simulink model "UGV"  (R2021b)
settings: Solver=VariableStepAuto  StartTime=0.0  StopTime=20  RelTol=1e-5
PreLoadFcn:
  | % initialize variables
  | initializeUnicycleModel;
undefined symbols (not defined in the file): ctrl, unicycle
settings Model: Creator=beniamino  LastModifiedBy=gioel
settings SolverCC: ZeroCrossAlgorithm=Adaptive
settings DataIOCC: InitialState=cartesianInitialStates  SaveFormat=Structure
settings DebuggingCC: IgnoredZcDiagnostic=none

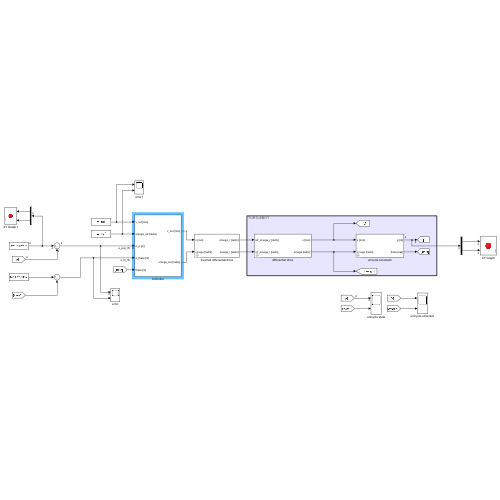
[thumbnail: Simulink's stored preview of the top-level diagram]
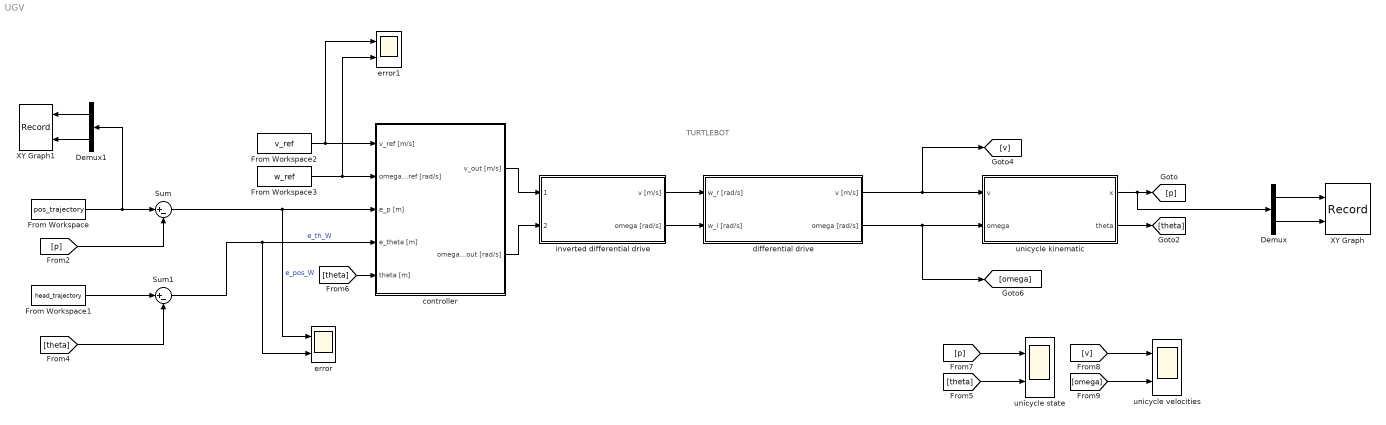
== system UGV ==
  note: TURTLEBOT
  Demux : Demux  Outputs=2
  Demux1 : Demux  Outputs=2
  From Workspace : FromWorkspace  VariableName=pos_trajectory
  From Workspace1 : FromWorkspace  VariableName=head_trajectory
  From Workspace2 : FromWorkspace  VariableName=v_ref
  From Workspace3 : FromWorkspace  VariableName=w_ref
  Sum : Sum  Inputs=|+-
  Sum1 : Sum  Inputs=|+-
  XY Graph : Record  FileSettingsInternal="{\"entries\":[{\"content\":{\"excelSettings\":{\"content\":{},\"type\":\"Streamout.ExcelSettings\"}},\"type\":\"Streamout.FileSettingStorage\",\"uuid\":\"13f76de6-499c-4140-b892-1cff53560195\"}],\"packageUris\":[\"http://schema.mathworks.com/mf0/streamout_blocks/R2020a\"],\"version\":\"1.0\"}"  Layout=[1 1]  SignalsInternal="{\"entries\":[{\"content\":{\"signals\":[{\"content\":{\"blockPath\":[\"UGV/XY Graph\"],\"channel\":[],\"dimensions\":[2],\"domain\":\"UGV/XY Graph\",\"hasChildren\":true,\"lineColor\":\"#77ac30\",\"plots\":[],\"port\":1,\"sid\":[\"\"],\"signalID\":231,\"signalName\":\"Mux\"},\"type\":\"RecordBlkView.Signal\",\"uuid\":\"fc620e12-1068-425f-97ba-d7612e3bfc5b\"},{\"content\":{\"blockPath\":[\"UGV/XY Graph\"],\"channel\":[1],\"dimensions\":[2],\"domain\":\"UGV/XY Graph\",\"lineColor\":\"#22b573\",\"parentID\":231,\"plots\":[],\"port\":1,\"sid\":[\"\"],\"signalID\":232,\"signalName\":\"Mux\"},\"type\":\"RecordBlkView.Signal\",\"uuid\":\"68e69acf-f8ce-4302-af24-f78098d05fbc\"},{\"content\":{\"blockPath\":[\"UGV/XY Graph\"],\"channel\":[],\"dimensions\":[2],\"domain\":\"UGV/XY Graph\",\"hasChildren\":true,\"lineColor\":\"#a2142f\",\"plots\":[],\"port\":2,\"sid\":[\"\"],\"signalID\":236,\"signalName\":\"Mux1\"},\"type\":\"RecordBlkView.Signal\",\"uuid\":\"04ece26b-ae12-44e9-b04e-33a75d772337\"},{\"content\":{\"blockPath\":[\"UGV/XY Graph\"],\"channel\":[1],\"dimensions\":[2],\"domain\":\"UGV/XY Graph\",\"lineColor\":\"#d95319\",\"parentID\":236,\"plots\":[],\"port\":2,\"sid\":[\"\"],\"signalID\":237,\"signalName\":\"Mux1\"},\"type\":\"RecordBlkView.Signal\",\"uuid\":\"c9d8e2c4-8b9b-40cc-9608-f78b40cf16be\"},{\"content\":{\"blockPath\":[\"UGV/XY Graph\"],\"channel\":[2],\"dimensions\":[2],\"domain\":\"UGV/XY Graph\",\"lineColor\":\"#edb120\",\"parentID\":231,\"plots\":[],\"port\":1,\"sid\":[\"\"],\"signalID\":240,\"signalName\":\"Mux\"},\"type\":\"RecordBlkView.Signal\",\"uuid\":\"41f5023c-efaf-446b-89f3-def201b5f8a6\"},{\"content\":{\"blockPath\":[\"UGV/XY Graph\"],\"channel\":[2],\"dimensions\":[2],\"domain\":\"UGV/XY Graph\",\"lineColor\":\"#7e2f8e\",\"parentID\":236,\"plots\":[],\"port\":2,\"sid\":[\"\"],\"signalID\":241,\"signalName\":\"Mux1\"},\"type\":\"RecordBlkView.Signal\",\"uuid\":\"77807980-b3eb-4829-a033-1b0bab4bfe93\"}]},\"type\":\"RecordBlkView.InputSignals\",\"uuid\":\"96da7dc8-515b-4996-b558-6921bb10ee03\"}],\"packageUris\":[\"http://schema.mathworks.com/mf0/streamout_blocks/R2020a\"],\"version\":\"1.0\"}"  VisualizationBindings="{\"xyplotplugin\":{\"info\":[{\"series\":[],\"subplotID\":1}]}}"  CompatibilityTag=XY
  XY Graph1 : Record  FileSettingsInternal="{\"entries\":[{\"content\":{\"excelSettings\":{\"content\":{},\"type\":\"Streamout.ExcelSettings\"}},\"type\":\"Streamout.FileSettingStorage\",\"uuid\":\"96a30333-0ed4-4420-9fea-70885ab511f6\"}],\"packageUris\":[\"http://schema.mathworks.com/mf0/streamout_blocks/R2020a\"],\"version\":\"1.0\"}"  Layout=[1 1]  SignalsInternal="{\"entries\":[{\"content\":{\"signals\":[]},\"type\":\"RecordBlkView.InputSignals\",\"uuid\":\"79161730-7756-4a65-8139-4cac527f2b4f\"}],\"packageUris\":[\"http://schema.mathworks.com/mf0/streamout_blocks/R2020a\"],\"version\":\"1.0\"}"  VisualizationBindings="{\"xyplotplugin\":{\"info\":[{\"series\":[{\"bindingParametersList\":[{\"parameter\":\"X-Axis\",\"signalID\":181,\"signalName\":\"Demux1:1\"},{\"parameter\":\"Y-Axis\",\"signalID\":185,\"signalName\":\"Demux1:2\"}],\"seriesID\":31783}],\"subplotID\":1}]}}"  CompatibilityTag=XY
  controller : Subsystem
  differential drive : Subsystem  mask(Differential drive for a unicycle){r=unicycle.diffDrive.r, d=unicycle.diffDrive.d, wheelDyEn=on, Tc=unicycle.diffDrive.Td, wheelsSpeedUpperLimit=unicycle.diffDrive.omegaWheelMax, wheelsSpeedLowerLimit=unicycle.diffDrive.omegaWheelMin}
      mask prompts: r "wheel radius"; d "interaxis lenght"; wheelDyEn "l.p.f. enable"; Tc "time constant [s]"; wheelsSpeedUpperLimit "max wheel speed  [rad/s]"; wheelsSpeedLowerLimit "min wheel speed [rad/s]"
      mask help:
      | Model of a differential drive.
      | It takes as input the derired wheel velocities and converts them to the corresponding driving velocity and stearing velocity.
      | Wheels dynamics can be taken into accont, along with output saturation.
      mask Help:
      | author: Beniamino Pozzan
      | email: beniamino.pozzan@phd.unipd.it
      mask Callback wheelDyEn:
      | % get the enable parameter
      | wheelDyEnStatus = get_param(gcb,'wheelDyEn');
      | enableStatus = get_param(gcb,'MaskEnables');
      | % if it is true, make Tc enabled
      | if strcmp(wheelDyEnStatus,'on')
      |     enableStatus{4}='on';
      | else
      |     enableStatus{4}='off';
      | end
      | set_param(gcb,'MaskEnables',enableStatus)
      mask TypeOptions wheelsSpeedUpperLimit: w_l saturator/UpperLimit | w_r saturator/UpperLimit
      mask TypeOptions wheelsSpeedLowerLimit: w_l saturator/LowerLimit | w_r saturator/LowerLimit
      mask DialogControl wheelDy Prompt: wheel dynamics
  error : Scope  NumInputPorts=2
  error1 : Scope  NumInputPorts=2
  inverted differential drive : Subsystem  mask(Inverted Differential drive for a unicycle){r=unicycle.diffDrive.r, d=unicycle.diffDrive.d}
      mask prompts: r "wheel radius"; d "interaxis lenght"
      mask help:
      | Inverted differential drive for a unicycle.
      | Provided the desired driving and stearing velocities, it computes the corresponding wheel velocities.
  unicycle kinematic : Subsystem  mask(Unicycle Kinematic Model){x0=unicycle.ic.x, y0=unicycle.ic.y, theta0=unicycle.ic.theta}
      mask prompts: x0 "x_0"; y0 "y_0"; theta0 "theta_0"
      mask help: kinematic model of a unicyle.
  unicycle state : Scope  NumInputPorts=2
  unicycle velocities : Scope  NumInputPorts=2
  wires:
  inverted differential drive/1(v [m/s]) -> differential drive/1(w_r [rad/s])
  inverted differential drive/2(omega [rad/s]) -> differential drive/2(w_l [rad/s])
  differential drive/1(v [m/s]) -> [v], unicycle kinematic/1(v)
  differential drive/2(omega [rad/s]) -> [omega], unicycle kinematic/2(omega)
  unicycle kinematic/1(x) -> Demux/1, [p]
  unicycle kinematic/2(theta) -> [theta]
  [p] -> Sum/2
  [theta] -> unicycle state/2
  [p] -> unicycle state/1
  [v] -> unicycle velocities/1
  [omega] -> unicycle velocities/2
  [theta] -> Sum1/2
  From Workspace1/1 -> Sum1/1
  controller/1(v_out [m/s]) -> inverted differential drive/1(1)
  controller/2(omega_out [rad/s]) -> inverted differential drive/2(2)
  Sum/1 -> error/1, controller/3(e_p [m])  "e_pos_W"
  Sum1/1 -> error/2, controller/4(e_theta [m])  "e_th_W"
  From Workspace2/1 -> error1/1, controller/1(v_ref [m/s])
  From Workspace3/1 -> error1/2, controller/2(omega_ref [rad/s])
  [theta] -> controller/5(theta [m])
  Demux/1 -> XY Graph/1
  Demux/2 -> XY Graph/2
  Demux1/1 -> XY Graph1/1
  From Workspace/1 -> Demux1/1, Sum/1
  Demux1/2 -> XY Graph1/2

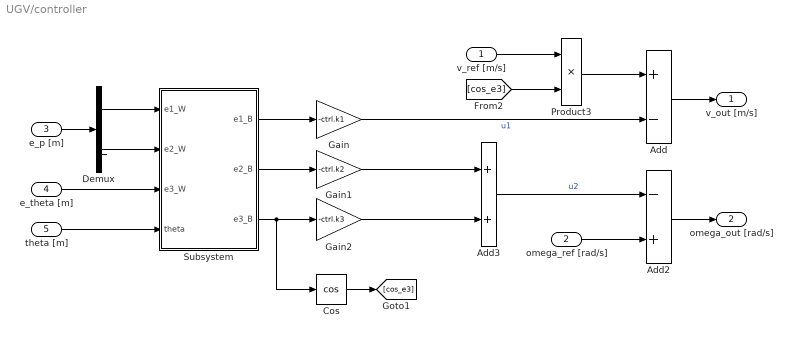
== system UGV/controller ==
  v_ref [m/s] : Inport
  omega_ref [rad/s] : Inport  Port=2
  e_p [m] : Inport  Port=3
  e_theta [m] : Inport  Port=4
  theta [m] : Inport  Port=5
  Add : Sum  Inputs=+-
  Add2 : Sum  Inputs=-+
  Add3 : Sum
  Cos : Trigonometry  Operator=cos
  Demux : Demux  Outputs=2
  Gain : Gain  Gain=-ctrl.k1
  Gain1 : Gain  Gain=-ctrl.k2
  Gain2 : Gain  Gain=-ctrl.k3
  Product3 : Product
  Subsystem : Subsystem
  v_out [m/s] : Outport
  omega_out [rad/s] : Outport  Port=2
  wires:
  e_p [m]/1 -> Demux/1
  Gain/1 -> Add/2  "u1"
  Gain1/1 -> Add3/1
  Gain2/1 -> Add3/2
  Subsystem/1(e1_B) -> Gain/1
  Subsystem/2(e2_B) -> Gain1/1
  Demux/1 -> Subsystem/1(e1_W)
  Demux/2 -> Subsystem/2(e2_W)
  e_theta [m]/1 -> Subsystem/3(e3_W)
  theta [m]/1 -> Subsystem/4(theta)
  Subsystem/3(e3_B) -> Cos/1, Gain2/1
  Cos/1 -> [cos_e3]
  v_ref [m/s]/1 -> Product3/1
  [cos_e3] -> Product3/2
  Add/1 -> v_out [m/s]/1
  Product3/1 -> Add/1
  omega_ref [rad/s]/1 -> Add2/2
  Add3/1 -> Add2/1  "u2"
  Add2/1 -> omega_out [rad/s]/1

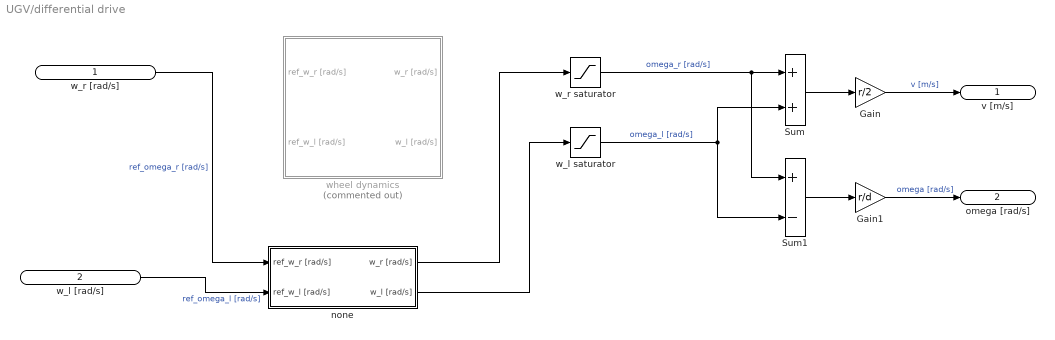
== system UGV/differential drive ==
  w_r [rad/s] : Inport  Unit=rad/s
  w_l [rad/s] : Inport  Port=2  Unit=rad/s
  Gain : Gain  Gain=r/2
  Gain1 : Gain  Gain=r/d
  Sum : Sum
  Sum1 : Sum  Inputs=+-
  none : Subsystem  VariantControl=wheelDyEn==false
  w_l saturator : Saturate  UpperLimit=wheelsSpeedUpperLimit  LowerLimit=wheelsSpeedLowerLimit
  w_r saturator : Saturate  UpperLimit=wheelsSpeedUpperLimit  LowerLimit=wheelsSpeedLowerLimit
  wheel dynamics : Subsystem  Commented=on  Variant=on
  v [m/s] : Outport  Unit=m/s
  omega [rad/s] : Outport  Port=2  Unit=rad/s
  wires:
  w_l saturator/1 -> Sum1/2, Sum/2  "omega_l [rad/s]"
  w_r saturator/1 -> Sum1/1, Sum/1  "omega_r [rad/s]"
  Gain1/1 -> omega [rad/s]/1  "omega [rad/s]"
  Sum1/1 -> Gain1/1
  Gain/1 -> v [m/s]/1  "v [m/s]"
  Sum/1 -> Gain/1
  w_r [rad/s]/1 -> none/1(ref_w_r [rad/s])  "ref_omega_r [rad/s]"
  w_l [rad/s]/1 -> none/2(ref_w_l [rad/s])  "ref_omega_l [rad/s]"
  none/1(w_r [rad/s]) -> w_r saturator/1
  none/2(w_l [rad/s]) -> w_l saturator/1

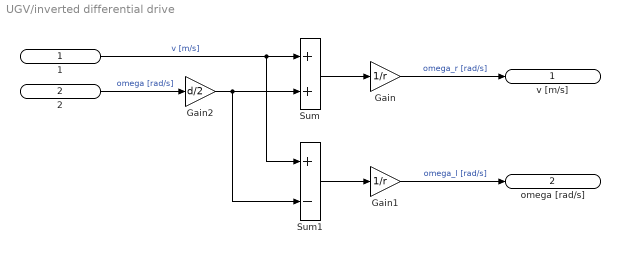
== system UGV/inverted differential drive ==
  1 : Inport  Unit=m/s
  2 : Inport  Port=2  Unit=rad/s
  Gain : Gain  Gain=1/r
  Gain1 : Gain  Gain=1/r
  Gain2 : Gain  Gain=d/2
  Sum : Sum
  Sum1 : Sum  Inputs=+-
  v [m/s] : Outport  Unit=rad/s
  omega [rad/s] : Outport  Port=2  Unit=rad/s
  wires:
  Gain2/1 -> Sum1/2, Sum/2
  Sum/1 -> Gain/1
  Gain/1 -> v [m/s]/1  "omega_r [rad/s]"
  Sum1/1 -> Gain1/1
  Gain1/1 -> omega [rad/s]/1  "omega_l [rad/s]"
  1/1 -> Sum1/1, Sum/1  "v [m/s]"
  2/1 -> Gain2/1  "omega [rad/s]"

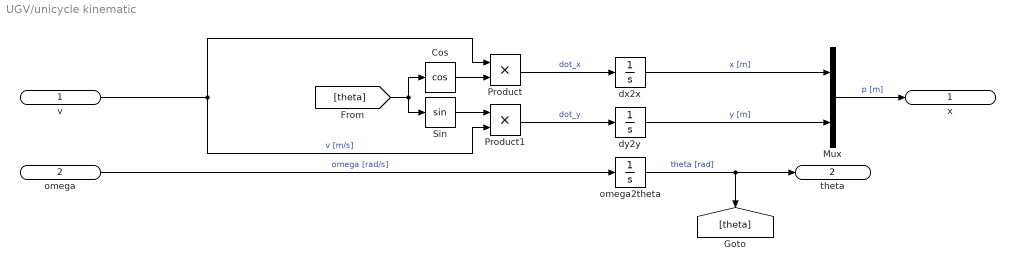
== system UGV/unicycle kinematic ==
  v : Inport  PortDimensions=1
  omega : Inport  Port=2  PortDimensions=1
  Cos : Trigonometry  Operator=cos
  Mux : Mux  Inputs=2
  Product : Product
  Product1 : Product
  Sin : Trigonometry
  dx2x : Integrator  InitialCondition=x0  ContinuousStateAttributes='pos_x'
  dy2y : Integrator  InitialCondition=y0  ContinuousStateAttributes='pos_y'
  omega2theta : Integrator  InitialCondition=theta0  ContinuousStateAttributes='theta'
  x : Outport  PortDimensions=2
  theta : Outport  Port=2  PortDimensions=1
  wires:
  Product1/1 -> dy2y/1  "dot_y"
  [theta] -> Sin/1, Cos/1
  v/1 -> Product/1, Product1/2  "v [m/s]"
  omega2theta/1 -> [theta], theta/1  "theta [rad]"
  omega/1 -> omega2theta/1  "omega [rad/s]"
  dy2y/1 -> Mux/2  "y [m]"
  Cos/1 -> Product/2
  dx2x/1 -> Mux/1  "x [m]"
  Sin/1 -> Product1/1
  Product/1 -> dx2x/1  "dot_x"
  Mux/1 -> x/1  "p [m]"

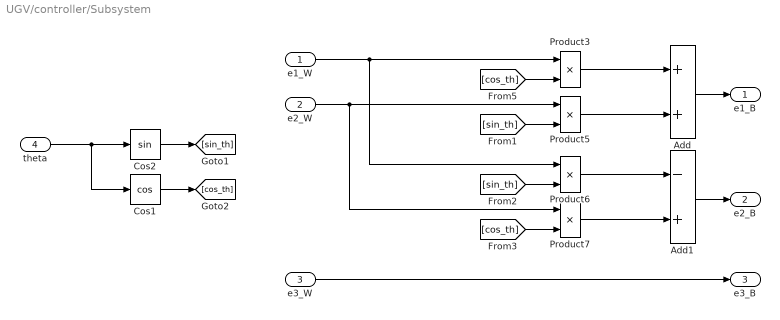
== system UGV/controller/Subsystem ==
  e1_W : Inport
  e2_W : Inport  Port=2
  e3_W : Inport  Port=3
  theta : Inport  Port=4
  Add : Sum
  Add1 : Sum  Inputs=-+
  Cos1 : Trigonometry  Operator=cos
  Cos2 : Trigonometry
  Product{3,5..7} (4 alike) : Product
  e1_B : Outport
  e2_B : Outport  Port=2
  e3_B : Outport  Port=3
  wires:
  Add/1 -> e1_B/1
  Add1/1 -> e2_B/1
  Cos2/1 -> [sin_th]
  Cos1/1 -> [cos_th]
  Product3/1 -> Add/1
  Product5/1 -> Add/2
  Product7/1 -> Add1/2
  Product6/1 -> Add1/1
  e1_W/1 -> Product6/1, Product3/1
  [cos_th] -> Product3/2
  e2_W/1 -> Product7/1, Product5/1
  [sin_th] -> Product5/2
  [sin_th] -> Product6/2
  [cos_th] -> Product7/2
  e3_W/1 -> e3_B/1
  theta/1 -> Cos1/1, Cos2/1

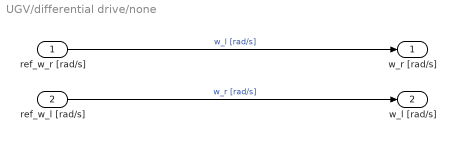
== system UGV/differential drive/none ==
  ref_w_r [rad/s] : Inport
  ref_w_l [rad/s] : Inport  Port=2
  w_r [rad/s] : Outport
  w_l [rad/s] : Outport  Port=2
  wires:
  ref_w_r [rad/s]/1 -> w_r [rad/s]/1  "w_l [rad/s]"
  ref_w_l [rad/s]/1 -> w_l [rad/s]/1  "w_r [rad/s]"

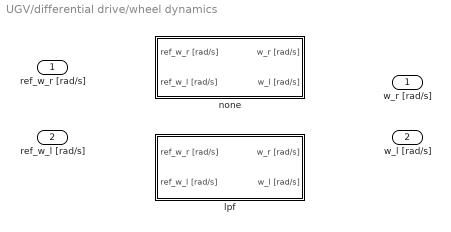
== system UGV/differential drive/wheel dynamics ==
  ref_w_r [rad/s] : Inport
  ref_w_l [rad/s] : Inport  Port=2
  lpf : Subsystem  VariantControl=wheelDyEn==true
  none : Subsystem  VariantControl=wheelDyEn==false
  w_r [rad/s] : Outport
  w_l [rad/s] : Outport  Port=2

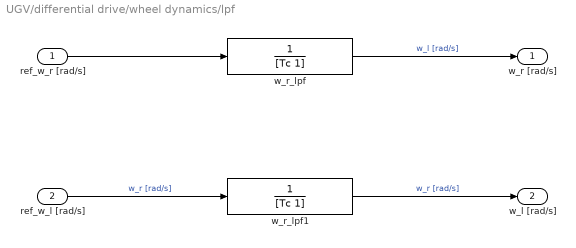
== system UGV/differential drive/wheel dynamics/lpf ==
  ref_w_r [rad/s] : Inport
  ref_w_l [rad/s] : Inport  Port=2
  w_r_lpf : TransferFcn  Denominator=[Tc 1]  ContinuousStateAttributes='w_r_lpf'
  w_r_lpf1 : TransferFcn  Denominator=[Tc 1]  ContinuousStateAttributes='w_r_lpf'
  w_r [rad/s] : Outport
  w_l [rad/s] : Outport  Port=2
  wires:
  ref_w_r [rad/s]/1 -> w_r_lpf/1
  w_r_lpf1/1 -> w_l [rad/s]/1  "w_r [rad/s]"
  w_r_lpf/1 -> w_r [rad/s]/1  "w_l [rad/s]"
  ref_w_l [rad/s]/1 -> w_r_lpf1/1  "w_r [rad/s]"

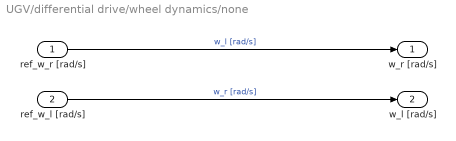
== system UGV/differential drive/wheel dynamics/none ==
  ref_w_r [rad/s] : Inport
  ref_w_l [rad/s] : Inport  Port=2
  w_r [rad/s] : Outport
  w_l [rad/s] : Outport  Port=2
  wires:
  ref_w_r [rad/s]/1 -> w_r [rad/s]/1  "w_l [rad/s]"
  ref_w_l [rad/s]/1 -> w_l [rad/s]/1  "w_r [rad/s]"
